simulink model "cic_filter_test_newnew_dec4_nonpoly_4"  (Simulink 7.4)
settings: Solver=ode45  StartTime=0.0  StopTime=10000  RelTol=1e-3
libraries: xbsIndex_r4 x213, simulink x3, xrbsComm_r4 x1, xps_library x1
(part 3 of 3)

== system cic_filter_test_newnew_dec4_nonpoly_4/npcic non-poly dec4/stage2/polynomial/shift_mult_array ==
  in : Inport
  sync : Inport  Port=2
  adder_tree2 : Subsystem
  delay1 : xbsIndex_r4/Delay  en=off  latency=1  dbl_ovrd=off  reg_retiming=off  block_type=delay
      settings: block_version=11.4
  shift2 : xbsIndex_r4/Shift  shift_dir=Left  shift_bits=1  en=off  latency=0  precision=User Defined  arith_type="Signed  (2's comp)"  n_bits=14  bin_pt=3  quantization=Truncate  overflow=Wrap  dbl_ovrd=off  block_type=shift
  sync_delay : xbsIndex_r4/Delay  en=off  latency=1  dbl_ovrd=off  reg_retiming=off  block_type=delay
      settings: block_version=11.4
  out1 : Outport
  out2 : Outport  Port=2
  out3 : Outport  Port=3
  out4 : Outport  Port=4
  sync_out : Outport  Port=5
  wires:
  in/1 -> delay1/1, adder_tree2/1(sync), shift2/1, adder_tree2/2(din_1)  "adder_trees_out1"
  adder_tree2/2(dout) -> out3/1, out2/1  "out2"
  delay1/1 -> out1/1, out4/1  "out1"
  sync/1 -> sync_delay/1
  shift2/1 -> adder_tree2/3(din_2)  "shift_out2"
  sync_delay/1 -> sync_out/1

== system cic_filter_test_newnew_dec4_nonpoly_4/npcic non-poly dec4/stage1/polynomial/shift_mult_array/adder_tree2 ==
  sync : Inport
  din_1 : Inport  Port=2
  din_2 : Inport  Port=3
  adder_0 : xbsIndex_r4/AddSub  mode=Addition  use_carryin=off  use_carryout=off  en=off  latency=1  precision=Full  arith_type=Unsigned  n_bits=16  bin_pt=14  quantization="Round  (unbiased: +/- Inf)"  overflow=Saturate  dbl_ovrd=off  use_behavioral_HDL=on  hw_selection=Fabric  pipelined=off  block_type=addsub
  sync_delay : xbsIndex_r4/Delay  en=off  latency=1  dbl_ovrd=off  reg_retiming=off  block_type=delay
      settings: block_version=11.4
  zero_in : xbsIndex_r4/Constant  arith_type=Unsigned  const=0  n_bits=18  bin_pt=17  explicit_period=off  period=1  equ=P=C  opselect=C  inp2=PCIN>>17  opr=+  inp1=P  carry=CIN  dbl_ovrd=off  block_type=constant
      settings: block_version=11.4
  sync_out : Outport
  dout : Outport  Port=2
  wires:
  din_1/1 -> adder_0/2
  sync_delay/1 -> sync_out/1
  sync/1 -> sync_delay/1
  din_2/1 -> adder_0/1
  adder_0/1 -> dout/1

== system cic_filter_test_newnew_dec4_nonpoly_4/npcic non-poly dec4/stage2/polynomial/shift_mult_array/adder_tree2 ==
  sync : Inport
  din_1 : Inport  Port=2
  din_2 : Inport  Port=3
  adder_0 : xbsIndex_r4/AddSub  mode=Addition  use_carryin=off  use_carryout=off  en=off  latency=1  precision=Full  arith_type=Unsigned  n_bits=16  bin_pt=14  quantization="Round  (unbiased: +/- Inf)"  overflow=Saturate  dbl_ovrd=off  use_behavioral_HDL=on  hw_selection=Fabric  pipelined=off  block_type=addsub
  sync_delay : xbsIndex_r4/Delay  en=off  latency=1  dbl_ovrd=off  reg_retiming=off  block_type=delay
      settings: block_version=11.4
  zero_in : xbsIndex_r4/Constant  arith_type=Unsigned  const=0  n_bits=18  bin_pt=17  explicit_period=off  period=1  equ=P=C  opselect=C  inp2=PCIN>>17  opr=+  inp1=P  carry=CIN  dbl_ovrd=off  block_type=constant
      settings: block_version=11.4
  sync_out : Outport
  dout : Outport  Port=2
  wires:
  din_1/1 -> adder_0/2
  sync_delay/1 -> sync_out/1
  sync/1 -> sync_delay/1
  din_2/1 -> adder_0/1
  adder_0/1 -> dout/1
